simulink model "SCPI_gain"  (R2025b)
settings: Solver=VariableStepAuto  StartTime=0.0  StopTime=inf  RelTol=1e-3
libraries: slpidlib x1
settings Model: Creator=Student13  LastModifiedBy=Student13

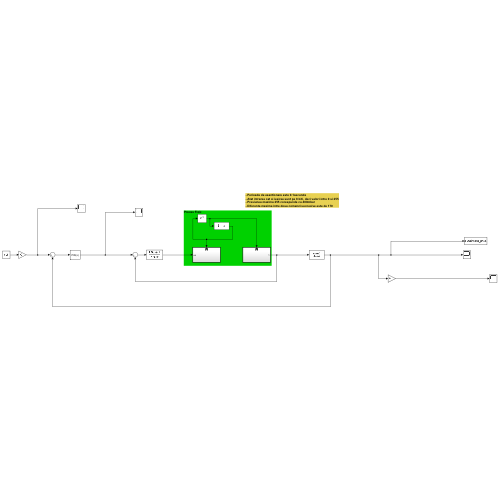
[thumbnail: Simulink's stored preview of the top-level diagram]
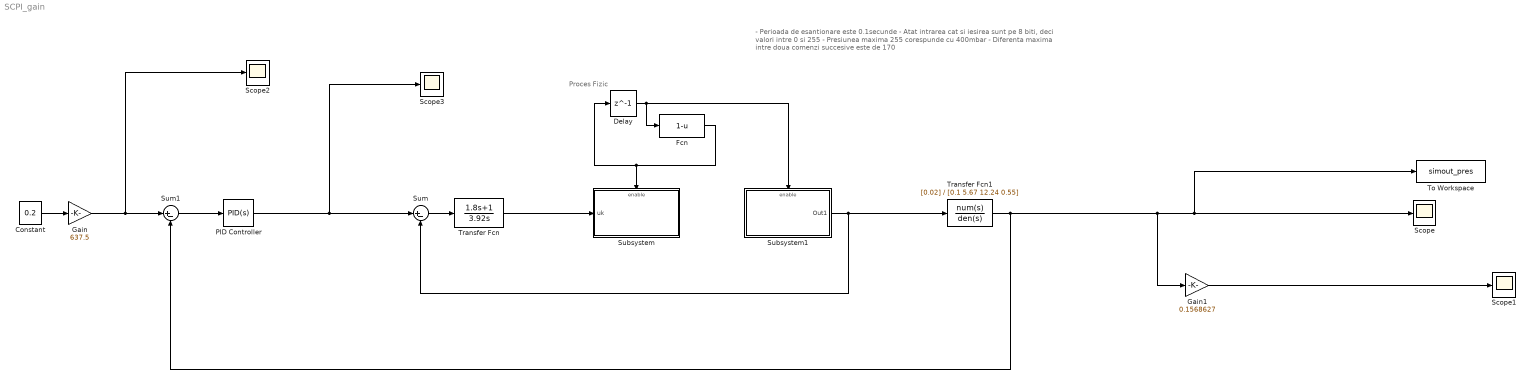
== system SCPI_gain ==
  note: Proces Fizic
  note: - Perioada de esantionare este 0.1secunde
      | - Atat intrarea cat si iesirea sunt pe 8 biti, deci valori intre 0 si 255
      | - Presiunea maxima 255 corespunde cu 400mbar
      | - Diferenta maxima intre doua comenzi succesive este de 170
  Constant : Constant  Value=0.2  OutDataTypeStr=double  SampleTime=0.1
  Delay : Delay  DelayLength=1  InitialCondition=0  SampleTime=0.05
  Fcn : Fcn  Expr=1-u
  Gain : Gain  Gain=637.5
  Gain1 : Gain  Gain=0.1568627
  PID Controller : slpidlib/PID Controller  Controller=PID  Form=Parallel  TimeDomain=Continuous-time  UseExternalTs=off  SampleTime=-1  IntegratorMethod=Forward Euler  FilterMethod=Forward Euler  ControllerParametersSource=internal  P=51.1  I=3.6943  UseKiTs=off  D=44.99  UseExternalDerivativeSource=off  N=10.53  UseFilter=on  TunerSelectOption=Transfer Function Based (PID Tuner App)  InitialConditionSource=internal  InitialConditionForIntegrator=0  InitialConditionForFilter=0  DifferentiatorICPrevScaledInput=0  ExternalReset=none  TrackingMode=off  Kt=1  LimitOutput=off  SatLimitsSource=internal  UpperSaturationLimit=inf  LowerSaturationLimit=-inf  LinearizeAsGain=on  AntiWindupMode=none  Kb=1  LimitIntegrator=off  UpperIntegratorSaturationLimit=inf  LowerIntegratorSaturationLimit=-inf  POutMin=[]  POutMax=[]  IOutMin=[]  IOutMax=[]  DOutMin=[]  DOutMax=[]  NOutMin=[]  NOutMax=[]  SumOutMin=[]  SumOutMax=[]  SaturationOutMin=[]  SaturationOutMax=[]  PParamMin=[]  PParamMax=[]  IParamMin=[]  IParamMax=[]  DParamMin=[]  DParamMax=[]  NParamMin=[]  NParamMax=[]  KbParamMin=[]  KbParamMax=[]  KtParamMin=[]  KtParamMax=[]  KbOutMin=[]  KbOutMax=[]  KtOutMin=[]  KtOutMax=[]  IntegratorOutMin=[]  IntegratorOutMax=[]  FilterOutMin=[]  FilterOutMax=[]  SumI1OutMin=[]  SumI1OutMax=[]  SumI2OutMin=[]  SumI2OutMax=[]  SumI3OutMin=[]  SumI3OutMax=[]  SumI4OutMin=[]  SumI4OutMax=[]  SumDOutMin=[]  SumDOutMax=[]  DifferentiatorOutMin=[]  DifferentiatorOutMax=[]  FilterDiffOutCoefMin=[]  FilterDiffOutCoefMax=[]  ReciprocalOutMin=[]  ReciprocalOutMax=[]  SumDenOutMin=[]  SumDenOutMax=[]  SumNumOutMin=[]  SumNumOutMax=[]  DivideOutMin=[]  DivideOutMax=[]  UdiffTsProdOutMin=[]  UdiffTsProdOutMax=[]  NTsProdOutMin=[]  NTsProdOutMax=[]  UintegralTsProdOutMin=[]  UintegralTsProdOutMax=[]  UngainTsProdOutMin=[]  UngainTsProdOutMax=[]  ClampingZeroOutDataTypeStr=Inherit: Inherit via back propagation  ClampingZeroOutMin=[]  ClampingZeroOutMax=[]  FilterDenConstantOutDataTypeStr=Inherit: Inherit via back propagation  FilterDenConstantOutMin=[]  FilterDenConstantOutMax=[]  PCopyOutDataTypeStr=Inherit: Inherit via back propagation  PCopyOutMin=[]  PCopyOutMax=[]  NCopyOutDataTypeStr=Inherit: Inherit via back propagation  NCopyOutMin=[]  NCopyOutMax=[]  IntegratorContinuousStateAttributes=''  IntegratorStateMustResolveToSignalObject=off  IntegratorRTWStateStorageClass=Auto  FilterContinuousStateAttributes=''  FilterStateMustResolveToSignalObject=off  FilterRTWStateStorageClass=Auto  ParallelPVariant=InternalParameters  IdealPVariant=Disabled  IVariant=InternalParameters  DVariant=InternalParameters  IntegratorVariant=Continuous  SatVariant=Disabled  AWVariant=Passthrough  PCopyVariant=Disabled  TRVariant=Disabled  FdbkBlocksVariant=Forward  IdealPFdbkVariant=Disabled  SatFdbkVariant=Disabled  DerivativeFilterVariant=ContFilter  NVariant=InternalParameters  NCopyVariant=Disabled  FilterICVariant=InternalICsFilter  IntegratorICVariant=InternalICs  ExternalResetVariant=Disabled  TRSumVariant=Passthrough  SumFdbkVariant=Disabled  SumVariant=Sum_PID  TsampFilterVariant=InternalTs  TsampNgainVariant=Passthrough  TsampIntegralVariant=Disabled_SignalSpec  ExternalSaturationOutDataTypeStr=Inherit: Same as second input  DerivativeSourceVariant=ErrorSignal  PreIntVariant=InternalPreInt
  Scope{,1..3} (4 alike) : Scope
      Scope settings: ActiveDisplayYMinimum=-54.10320475322078  ActiveDisplayYMaximum=182.62964830320931
      Scope2 settings: DataLoggingVariableName=ScopeData2
      Scope3 settings: DataLoggingVariableName=ScopeData3
  Subsystem : Subsystem
  Subsystem1 : Subsystem
  Sum : Sum  Inputs=|+-
  Sum1 : Sum  Inputs=|+-
  To Workspace : ToWorkspace  VariableName=simout_pres  SaveFormat=Timeseries  SampleTime=0.1
  Transfer Fcn : TransferFcn  Numerator=[1.8 1]  Denominator=[3.92 0]
  Transfer Fcn1 : TransferFcn  Numerator=[0.02]  Denominator=[0.1 5.67 12.24 0.55]
  wires:
  PID Controller/1 -> Scope3/1, Sum/1
  Gain/1 -> Scope2/1, Sum1/1
  Transfer Fcn1/1 -> To Workspace/1, Scope/1, Gain1/1, Sum1/2
  Gain1/1 -> Scope1/1
  Sum1/1 -> PID Controller/1
  Constant/1 -> Gain/1
  Transfer Fcn/1 -> Subsystem/1(uk)
  Delay/1 -> Fcn/1, Subsystem1/Enable
  Subsystem1/1(Out1) -> Transfer Fcn1/1, Sum/2
  Fcn/1 -> Delay/1, Subsystem/Enable
  Sum/1 -> Transfer Fcn/1

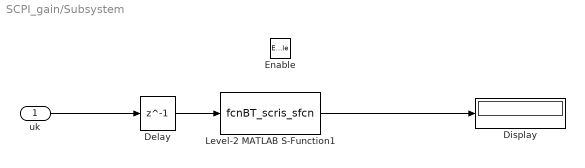
== system SCPI_gain/Subsystem ==
  uk : Inport
  Enable : EnablePort
  Delay : Delay  DelayLength=1  SampleTime=0.1
  Display : Display
  Level-2 MATLAB S-Function1 : M-S-Function  FunctionName=fcnBT_scris_sfcn
  wires:
  Level-2 MATLAB S-Function1/1 -> Display/1
  uk/1 -> Delay/1
  Delay/1 -> Level-2 MATLAB S-Function1/1

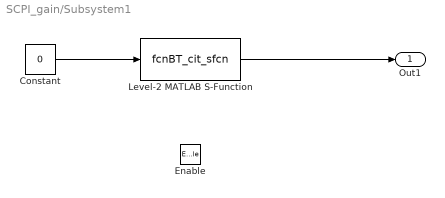
== system SCPI_gain/Subsystem1 ==
  Enable : EnablePort
  Constant : Constant  Value=0
  Level-2 MATLAB S-Function : M-S-Function  FunctionName=fcnBT_cit_sfcn
  Out1 : Outport  VectorParamsAs1DForOutWhenUnconnected=off
  wires:
  Level-2 MATLAB S-Function/1 -> Out1/1
  Constant/1 -> Level-2 MATLAB S-Function/1
